simulink model "full_model"  (R2017a)
settings: Solver=ode15s  StartTime=0.0  StopTime=40  FixedStep=0.0000001  RelTol=1e-3
undefined symbols (not defined in the file): AUV, HydroDyn, kc, Path, Vfwd, Vz, Z_delay
libraries: simulink x4, simulink_extras x1
settings Model: Creator=Eugene  LastModifiedBy=corsair
settings DebuggingCC: ParameterOverflowMsg=warning
settings HardwareCC: ProdHWDeviceType=AMD->x86-64 (Windows64)

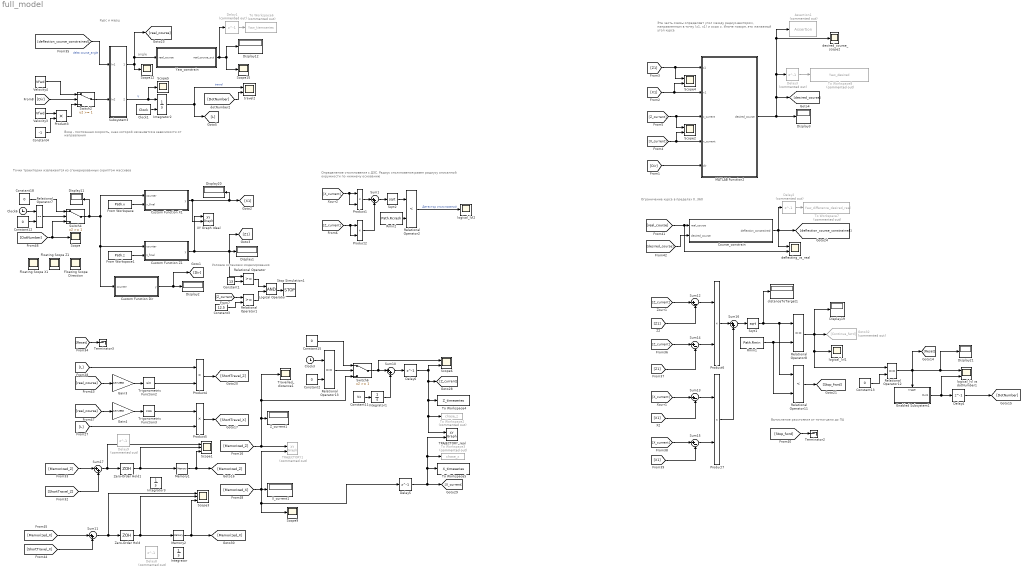
== system full_model ==
  note: Условие остановки моделирования
  note: Ограничение курса в пределах 0..360
  note: Определение столкновения с ДЗС. Радиус столкновения равен радиусу описанной окружности по нижнему основанию
  note: Точки траектории извлекаются из сгенерированных скриптом массивов
  note: Вход - постоянная скорость, знак которой изменяется в зависимости от направления
  note: Курс и марш
  note: Вычисление расстояния от точки-цели до ПА
  note: angle
  note: Эта часть схемы определяет угол между радиус-вектором, направленным в точку (z1, x1) и осью z. Иначе говоря, это желаемый угол курса
  Assertion1 : Assertion  Commented=on  AssertionFailFcn=-1
  Clock1 : simulink_extras/Flip Flops/Clock  period=Z_delay
  Clock3 : Clock
  Clock6 : Clock
  Constant1 : Constant  Value=13
  Constant11 : Constant  Value=Vz
  Constant{2,12..13,15,18} (5 alike) : Constant  Value=0
  Constant3 : Constant  Value=12.5
  Constant4 : Constant  Value=-1
  Course_constrain : MATLAB Function  TreatAsAtomicUnit=on
  Custom Function Dir : MATLAB Function  TreatAsAtomicUnit=on
  Custom Function X1 : MATLAB Function  TreatAsAtomicUnit=on
  Custom Function Z1 : MATLAB Function  TreatAsAtomicUnit=on
  Delay1 : Delay  Commented=on  DelayLength=1  InitialCondition=180  SampleTime=Z_delay
  Delay2 : Delay  Commented=on  DelayLength=1  InitialCondition=0  SampleTime=Z_delay
  Delay3 : Delay  Commented=on  DelayLength=1  InitialCondition=15  SampleTime=Z_delay
  Delay4 : Delay  DelayLength=1  InitialCondition=0  SampleTime=Z_delay
  Delay5 : Delay  DelayLength=1  InitialCondition=15  SampleTime=Z_delay
  Delay6 : Delay  DelayLength=1  SampleTime=Z_delay
  Delay8 : Delay  Commented=on  DelayLength=1  InitialCondition=15
  Delay9 : Delay  Commented=on  DelayLength=1
  Display{1..3,11..12,19..21} (8 alike) : Display
  Enabled Subsystem1 : Subsystem  TreatAsAtomicUnit=on
  Floating Scope Direction : Scope
      settings: Floating=on
  Floating Scope X1 : Scope
      settings: Floating=on
  Floating Scope Z1 : Scope
      settings: Floating=on
  From Workspace : FromWorkspace  VariableName=Path.x
  From Workspace1 : FromWorkspace  VariableName=Path.z
  Gain3 : Gain  Gain=1/57.2958
  Gain4 : Gain  Gain=1/57.2958
  Goto32 : Goto  Commented=on  GotoTag=Continue_fwrd
  Integrator : Integrator  InitialCondition=15
  Integrator1 : Integrator
  Integrator2 : Integrator  ExternalReset=rising
  Integrator3 : Integrator
  Logical Operator : Logic  AllPortsSameDT=off  OutDataTypeStr=boolean
  MATLAB Function2 : MATLAB Function  TreatAsAtomicUnit=on
  Memory1 : Memory  InheritSampleTime=on  LinearizeMemory=on
  Memory2 : Memory  X0=15  InheritSampleTime=on  LinearizeMemory=on
  Product{1..7} (7 alike) : Product
  Relational Operator : RelationalOperator  OutDataTypeStr=boolean  RndMeth=Simplest
  Relational Operator1 : RelationalOperator  OutDataTypeStr=boolean  RndMeth=Simplest
  Relational Operator11 : RelationalOperator  Operator=<  OutDataTypeStr=boolean  RndMeth=Simplest
  Relational Operator12 : RelationalOperator  Operator===  OutDataTypeStr=boolean  RndMeth=Simplest
  Relational Operator13 : RelationalOperator  Operator===  OutDataTypeStr=boolean  RndMeth=Simplest
  Relational Operator2 : RelationalOperator  Operator=<  OutDataTypeStr=boolean  RndMeth=Simplest
  Relational Operator7 : RelationalOperator  Operator===  OutDataTypeStr=boolean  RndMeth=Simplest
  Relational Operator8 : RelationalOperator  OutDataTypeStr=boolean  RndMeth=Simplest
  Rmin1 : Constant  Value=Path.Rmin
  Rmin2 : Constant  Value=Path.Rcrash
  Scope{,5,9,12,15} (5 alike) : Scope
  Scope1 : Scope  NumInputPorts=3
  Scope2 : Scope  NumInputPorts=2
  Scope3 : Scope  NumInputPorts=3
  Scope4 : Scope  NumInputPorts=2
  Scope6 : Scope  NumInputPorts=2
  Sqrt1 : Sqrt  SaturateOnIntegerOverflow=on
  Sqrt2 : Sqrt  SaturateOnIntegerOverflow=on
  Stop Simulation1 : Stop
  Subsystem3 : Subsystem
  Sum{1,10..11,16..17} (5 alike) : Sum  Inputs=|++
  Sum{12..15} (4 alike) : Sum  Inputs=|+-
  Switch2 : Switch  Threshold=1
  Switch4 : Switch  Threshold=1
  Switch6 : Switch  Threshold=1
  TRAJECTORY1 : simulink/Sinks/XY Graph  Commented=on  xmin=-15  xmax=15  ymin=-15  ymax=15  st=-1
  TRAJECTORY_real : simulink/Sinks/XY Graph  xmin=-15  xmax=15  ymin=-15  ymax=15  st=-1
  Terminator2 : Terminator
  Terminator3 : Terminator
  To Workspace2 : ToWorkspace  Commented=on  VariableName=chase_z  SampleTime=-1
  To Workspace3 : ToWorkspace  Commented=on  VariableName=chase_x  SampleTime=-1
  To Workspace4 : ToWorkspace  VariableName=Z_timeseries  SaveFormat=Timeseries  SampleTime=-1
  To Workspace5 : ToWorkspace  VariableName=X_timeseries  SaveFormat=Timeseries  SampleTime=-1
  To Workspace6 : ToWorkspace  Commented=on  VariableName=Yaw_tiemseries  SaveFormat=Timeseries  SampleTime=-1
  To Workspace7 : ToWorkspace  Commented=on  VariableName=Yaw_difference_desired_real  SaveFormat=Timeseries  SampleTime=-1
  To Workspace8 : ToWorkspace  Commented=on  VariableName=Yaw_desired  SaveFormat=Timeseries  SampleTime=-1
  Travelled_distance1 : Scope
  Trigonometric Function2 : Trigonometry
  Trigonometric Function3 : Trigonometry  Operator=cos
  Velocity3 : Constant  Value=Vfwd
  Velocity4 : Constant  Value=Vfwd
  XY Graph Ideal : simulink/Sinks/XY Graph  xmin=-15  xmax=15  ymin=-15  ymax=15  st=-1
  X_current1 : Display
  Yaw_constrain : MATLAB Function  TreatAsAtomicUnit=on
  Z_current1 : Display
  Zero-Order Hold : ZeroOrderHold  SampleTime=0.033
  Zero-Order Hold1 : ZeroOrderHold  SampleTime=0.033
  deflecting_vs_real : Scope  NumInputPorts=2
  desired_course_scope2 : Scope
  distanceToTarget1 : Display
  logical_lvl vs dotNumber1 : Scope  NumInputPorts=2
  logical_lvl1 : Scope
  logical_lvl2 : Scope
  travel2 : Scope  NumInputPorts=2
  wires:
  Switch4/1 -> Custom Function Dir/1(counter), Custom Function Z1/1(counter), Custom Function X1/1(counter), Display11/1
  Sum14/1 -> Product6/2
  [Stop_fwrd] -> Terminator2/1
  Clock6/1 -> Relational Operator7/1
  Delay6/1 -> To Workspace4/1, TRAJECTORY_real/1, To Workspace2/1, [Z_current], Scope6/2
  [Reset] -> Terminator3/1
  Constant18/1 -> Switch4/1
  Relational Operator7/1 -> Switch4/2
  [real_course] -> deflecting_vs_real/2, Course_constrain/1(real_course)
  Course_constrain/1(deflection_constrained) -> Delay2/1, deflecting_vs_real/1, [deflection_course_constrained]
  [real_course] -> Gain3/1
  Yaw_constrain/1(real_course_out) -> Delay1/1, Scope15/1, Display12/1
  Constant12/1 -> Relational Operator7/2
  Switch6/1 -> Scope6/1, Sum10/1
  Memory2/1 -> Scope3/3, [Memorized_X]
  Product4/1 -> [ShortTravel_Z]
  [ShortTravel_X] -> Sum11/2
  Sum13/1 -> Product7/1
  Trigonometric Function2/1 -> Product4/2
  [Z1] -> Sum14/2
  [Z_current] -> Sum14/1
  [X1] -> Sum13/2
  [Z_current] -> Sum12/1
  [L] -> Product4/1
  Gain3/1 -> Trigonometric Function2/1
  Sum12/1 -> Product6/1
  Delay4/1 -> [DotNumber]
  Sum15/1 -> Product7/2
  Product7/1 -> Sum16/2
  Constant15/1 -> Switch6/1
  Custom Function X1/1(y) -> Display20/1, [X1], XY Graph Ideal/2
  Constant13/1 -> Relational Operator12/2
  Relational Operator12/1 -> [Reset], Enabled Subsystem1/Trigger, logical_lvl vs dotNumber1/1, Display21/1
  [X_current] -> Sum15/1
  Subsystem3/1(Out1) -> [real_course], Yaw_constrain/1(real_course), Scope12/1
  Relational Operator11/1 -> [Stop_fwrd]
  Integrator1/1 -> Sum10/2
  Rmin1/1 -> Relational Operator8/2, Relational Operator11/2
  [X1] -> Sum15/2
  Sum16/1 -> Sqrt1/1
  [X_current] -> Sum13/1
  [Memorized_Z] -> Sum17/1
  [DotNumber] -> Scope/1, Switch4/3
  [Memorized_Z] -> Switch6/3, Travelled_distance1/1, Z_current1/1, TRAJECTORY1/1
  [Z1] -> Sum12/2
  Constant2/1 -> Relational Operator13/2
  Custom Function Z1/1(y) -> Relational Operator/1, Display1/1, [Z1], XY Graph Ideal/1
  Product6/1 -> Sum16/1
  [ShortTravel_Z] -> Sum17/2
  [deflection_course_constrained] -> Subsystem3/1(In1)  "delta course_angle"
  Gain4/1 -> Trigonometric Function3/1
  [L] -> Product5/2
  [desired_course] -> Course_constrain/2(desired_course)
  Sum10/1 -> Delay6/1
  Clock3/1 -> Relational Operator13/1
  Product5/1 -> [ShortTravel_X]
  Delay5/1 -> [X_current], To Workspace5/1, TRAJECTORY_real/2, To Workspace3/1
  [Memorized_X] -> Sum11/1
  Enabled Subsystem1/1(Out1) -> Delay4/1, logical_lvl vs dotNumber1/2
  Relational Operator13/1 -> Switch6/2
  [Memorized_X] -> Scope9/1, Delay5/1, TRAJECTORY1/2, X_current1/1
  Trigonometric Function3/1 -> Product5/1
  Relational Operator8/1 -> Display19/1, Relational Operator12/1, logical_lvl1/1, Goto32/1
  [real_course] -> Gain4/1
  Memory1/1 -> Scope1/3, [Memorized_Z]
  Constant11/1 -> Integrator1/1
  Sqrt1/1 -> Relational Operator8/1, Relational Operator11/1, distanceToTarget1/1
  Custom Function Dir/1(y) -> Display2/1, [Dir]
  [Dir] -> MATLAB Function2/5(dir)
  [Z1] -> Scope4/1, MATLAB Function2/1(z1)
  [Z_current] -> MATLAB Function2/3(z_current), Scope2/1
  [X1] -> MATLAB Function2/2(x1), Scope4/2
  [X_current] -> Scope2/2, MATLAB Function2/4(x_current)
  From Workspace/1 -> Custom Function X1/2(x_final)
  From Workspace1/1 -> Custom Function Z1/2(z_final)
  Delay1/1 -> To Workspace6/1
  Delay2/1 -> To Workspace7/1
  Delay3/1 -> To Workspace8/1
  MATLAB Function2/1(desired_course) -> Assertion1/1, desired_course_scope2/1, Delay3/1, [desired_course], Display3/1
  [X_current] -> Product1/2, Product1/1
  [Z_current] -> Product2/2, Product2/1
  Product1/1 -> Sum1/1
  Product2/1 -> Sum1/2
  Sum1/1 -> Sqrt2/1
  Sqrt2/1 -> Relational Operator2/1
  Relational Operator2/1 -> logical_lvl2/1  "Детектор столкновений"
  Rmin2/1 -> Relational Operator2/2
  Relational Operator/1 -> Logical Operator/1
  Constant1/1 -> Relational Operator/2
  Constant3/1 -> Relational Operator1/2
  [Z_current] -> Relational Operator1/1
  Relational Operator1/1 -> Logical Operator/2
  Logical Operator/1 -> Stop Simulation1/1
  Constant4/1 -> Product3/2
  Product3/1 -> Switch2/3
  Velocity3/1 -> Product3/1
  Velocity4/1 -> Switch2/1
  [Dir] -> Switch2/2
  Switch2/1 -> Subsystem3/2(In2)
  Clock1/1 -> Integrator2/2
  Integrator2/1 -> [L], travel2/1  "travel"
  [DotNumber] -> travel2/2
  Subsystem3/2(Out2) -> Scope5/1, Integrator2/1  "V"
  Zero-Order Hold/1 -> Memory2/1, Scope3/2
  Sum11/1 -> Zero-Order Hold/1, Scope3/1
  Sum17/1 -> Zero-Order Hold1/1, Scope1/1
  Zero-Order Hold1/1 -> Memory1/1, Scope1/2

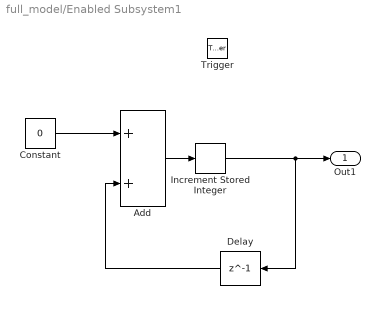
== system full_model/Enabled Subsystem1 ==
  Trigger : TriggerPort  VariantControl=Variant  PortDimensions=1
  Add : Sum
  Constant : Constant  Value=0
  Delay : Delay  DelayLength=1  InitialCondition=0
  Increment Stored Integer : simulink/Additional Math & Discrete/Additional Math: Increment - Decrement/Increment Stored Integer
  Out1 : Outport
  wires:
  Constant/1 -> Add/1
  Delay/1 -> Add/2
  Add/1 -> Increment Stored Integer/1
  Increment Stored Integer/1 -> Delay/1, Out1/1

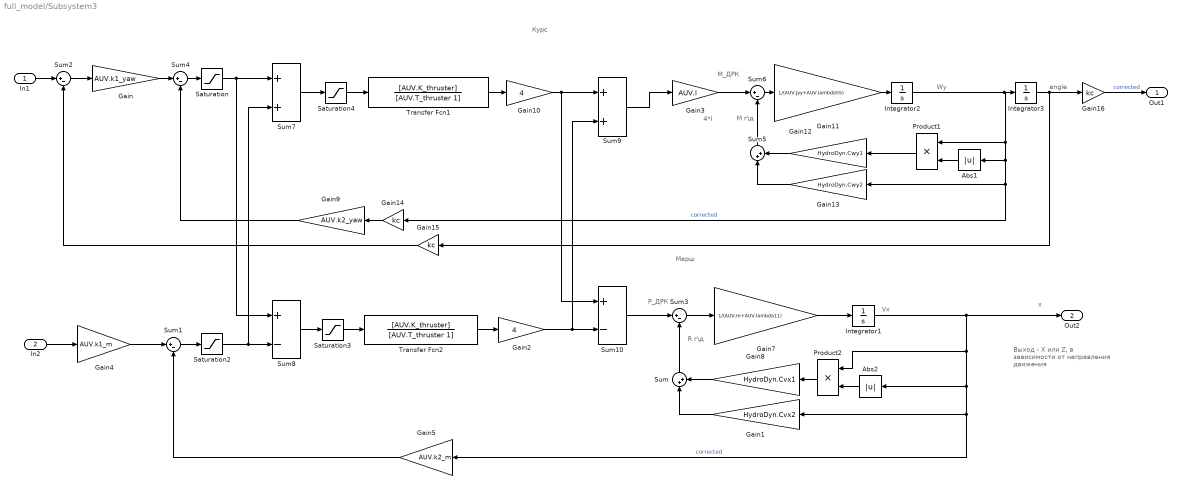
== system full_model/Subsystem3 ==
  note: Курс
  note: Wy
  note: M_ДРК
  note: 4*l
  note: angle
  note: M г\д
  note: Марш
  note: x
  note: R г\д
  note: P_ДРК
  note: Vx
  note: Выход - X или Z, в зависимости от направления движения
  In1 : Inport
  In2 : Inport  Port=2
  Abs1 : Abs
  Abs2 : Abs
  Gain : Gain  Gain=AUV.k1_yaw
  Gain1 : Gain  Gain=HydroDyn.Cvx2
  Gain10 : Gain  Gain=4
  Gain11 : Gain  Gain=1/(AUV.Jyy+AUV.lambda55)
  Gain12 : Gain  Gain=HydroDyn.Cwy1
  Gain13 : Gain  Gain=HydroDyn.Cwy2
  Gain14 : Gain  Gain=kc
  Gain15 : Gain  Gain=kc
  Gain16 : Gain  Gain=kc
  Gain2 : Gain  Gain=4
  Gain3 : Gain  Gain=AUV.l
  Gain4 : Gain  Gain=AUV.k1_m
  Gain5 : Gain  Gain=AUV.k2_m
  Gain7 : Gain  Gain=1/(AUV.m+AUV.lambda11)
  Gain8 : Gain  Gain=HydroDyn.Cvx1
  Gain9 : Gain  Gain=AUV.k2_yaw
  Integrator1 : Integrator  InitialCondition=0.7
  Integrator2 : Integrator
  Integrator3 : Integrator  InitialCondition=3.1416
  Product1 : Product
  Product2 : Product
  Saturation : Saturate  UpperLimit=24  LowerLimit=-24
  Saturation2 : Saturate  UpperLimit=24  LowerLimit=-24
  Saturation3 : Saturate  UpperLimit=12  LowerLimit=-12
  Saturation4 : Saturate  UpperLimit=12  LowerLimit=-12
  Sum : Sum  Inputs=|++
  Sum{1..4,6} (5 alike) : Sum  Inputs=|+-
  Sum10 : Sum  Inputs=+-
  Sum5 : Sum  Inputs=|++
  Sum7 : Sum
  Sum8 : Sum  Inputs=+-
  Sum9 : Sum
  Transfer Fcn1 : TransferFcn  Numerator=[AUV.K_thruster]  Denominator=[AUV.T_thruster 1]
  Transfer Fcn2 : TransferFcn  Numerator=[AUV.K_thruster]  Denominator=[AUV.T_thruster 1]
  Out1 : Outport
  Out2 : Outport  Port=2
  wires:
  Gain12/1 -> Sum5/2
  Product1/1 -> Gain12/1
  Gain11/1 -> Integrator2/1
  Gain9/1 -> Sum4/2
  Gain/1 -> Sum4/1
  Transfer Fcn1/1 -> Gain10/1
  Sum6/1 -> Gain11/1
  Gain14/1 -> Gain9/1
  Gain15/1 -> Sum2/2
  Gain13/1 -> Sum5/1
  Abs1/1 -> Product1/2
  Sum5/1 -> Sum6/2
  Integrator2/1 -> Integrator3/1, Abs1/1, Gain14/1, Gain13/1, Product1/1  "corrected"
  Sum2/1 -> Gain/1
  Integrator3/1 -> Gain16/1, Gain15/1
  In1/1 -> Sum2/1
  Gain16/1 -> Out1/1  "corrected"
  Sum4/1 -> Saturation/1
  Integrator1/1 -> Gain5/1, Gain1/1, Abs2/1, Product2/1, Out2/1  "corrected"
  Sum1/1 -> Saturation2/1
  Gain7/1 -> Integrator1/1
  Sum3/1 -> Gain7/1
  Abs2/1 -> Product2/2
  Gain1/1 -> Sum/1
  Gain4/1 -> Sum1/1
  Gain8/1 -> Sum/2
  Transfer Fcn2/1 -> Gain2/1
  Sum/1 -> Sum3/2
  Gain5/1 -> Sum1/2
  In2/1 -> Gain4/1
  Product2/1 -> Gain8/1
  Saturation/1 -> Sum8/1, Sum7/1
  Sum7/1 -> Saturation4/1
  Saturation4/1 -> Transfer Fcn1/1
  Saturation2/1 -> Sum7/2, Sum8/2
  Sum8/1 -> Saturation3/1
  Saturation3/1 -> Transfer Fcn2/1
  Gain3/1 -> Sum6/1
  Gain10/1 -> Sum9/1, Sum10/1
  Sum9/1 -> Gain3/1
  Gain2/1 -> Sum9/2, Sum10/2
  Sum10/1 -> Sum3/1

== matlab function full_model/MATLAB Function2 ==
  data: z1 input; x1 input; z_current input; desired_course output; x_current input; dir input
function desired_course = fcn(z1, x1, z_current, x_current, dir)

delta_x = x1 - x_current;
delta_z = z1 - z_current;

%1
if (delta_x >= 0) && (delta_z >= 0)
    desired_course = 57.2958*atan(delta_z / delta_x);
%2    
elseif (delta_x >= 0) && (delta_z < 0)
    desired_course = 360 - 57.2958*atan( abs(delta_z) / delta_x);
%3    
elseif (delta_x < 0) && (delta_z < 0)    
    desired_course = 180 + 57.2958*atan(abs(delta_z) / abs(delta_x));
%4    
elseif (delta_x < 0) && (delta_z >= 0)    
    desired_course = 180 - 57.2958*atan( delta_z / abs(delta_x));   
    
else 
    desired_course = -1;
end

    
% При движении назад отнимаем от 360-и    
if dir == -1
    desired_course = desired_course - 180;
end
    
end

== matlab function full_model/Custom Function Dir ==
  data: counter input; y output
function y = fcn(counter)

%L = 1.76;
% 1 - fwd, -1 - backward

    if mod(int32(counter), 2) == 1
        y = 1;
    else
        y = -1;
    end
    
    % NB: по началу нужно двигаться 2 раза вперёд: от (0, 15) к (0, 13) и
    % далее к первой путевой точке
    if counter == 0
        y = 1;
    end
end

== matlab function full_model/Custom Function X1 ==
  data: counter input; y output; x_final input
function y = fcn( counter, x_final)

%L = 1.76;

    if counter > 0 && counter < 48
        y = x_final(counter);
    else
        y = 13;
    end

% switch counter
%     case 1
%       y = 5.75;
%     case 2
%       y = 12.56;
%     case 3
%       y = 5.36;
%     case 4
%       y = 11.26;
%     case 5
%       y = 4.6;
%     case 6
%       y = 9.19;
%     case 7
%       y = 3.53;
%      
%    otherwise
%       y = 13;
end

== matlab function full_model/Custom Function Z1 ==
  data: counter input; y output; z_final input
function y = fcn(counter, z_final)

%L = 1.76;

    if counter > 0 && counter < 48
        y = z_final(counter);
    else
        y = 0;
    end


% switch counter
%    
%     case 1
%       y = -0.76;
%     case 2
%         y = -3.36;
%     case 3
%       y = -2.22;
%     case 4
%       y = -6.5;
%     case 5
%       y = -3.53;
%     case 6
%       y = -9.19;
%     case 7
%         y = -4.6;
%    otherwise
%       y = 0;

end

== matlab function full_model/Yaw_constrain ==
  data: real_course input; real_course_out output
function real_course_out   = fcn(real_course)

    % Приводим к стандарту
    if real_course < 0
        real_course_out = 360 - abs(real_course);
    elseif real_course >= 360
        real_course_out = real_course - 360;
    else    
        real_course_out = real_course;
    end

end

== matlab function full_model/Course_constrain ==
  data: real_course input; desired_course input; deflection_constrained output
function deflection_constrained   = fcn(real_course, desired_course)

    % предстоит повернуться более чем на 180 градусов
    % текущее положение курса не имеет никакого значения,
    %важно лишь конечное положение.
    % Па должен поворачиват менее чем на 180 градусов
    
    if abs(desired_course - real_course) > 180
    % выполняем ограничение
        if desired_course > 180
            deflection_constrained = desired_course - 360;
        %elseif desired_course < -180
        %    deflection_constrained = 360 + desired_course;
        else
            deflection_constrained = desired_course;
        end
    % иначе просто приравниваем
    else
        deflection_constrained = desired_course;
    end
end
